simulink model "turtle_waypoint"  (R2017b)
settings: Solver=FixedStepDiscrete  StartTime=0.0  StopTime=inf  FixedStep=0.1  RelTol=1e-3  EnableMultiTasking=on
undefined symbols (not defined in the file): Angular, Linear
libraries: robotlib x3, simulink x1
settings Model: Creator=The MathWorks, Inc.  LastModifiedBy=mraudett
settings DataIOCC: LimitDataPoints=on  SaveFormat=Array
settings OptimizationCC: DefaultUnderspecifiedDataType=single  LifeSpan=1  MaxStackSize=64
settings DebuggingCC: SolverPrmCheckMsg=warning  SFUnexpectedBacktrackingDiag=warning  SFNoUnconditionalDefaultTransitionDiag=warning  SFExecutionAtInitializationDiag=none
settings HardwareCC: ProdBitPerPointer=32  ProdBitPerSizeT=32  ProdBitPerPtrDiffT=32  ProdLargestAtomicFloat=None  ProdIntDivRoundTo=Undefined  ProdEndianess=Unspecified  ProdWordSize=32  ProdHWDeviceType=Generic->Unspecified (assume 32-bit Generic)  TargetHWDeviceType=Generic->Unspecified (assume 32-bit Generic)  UseEmbeddedCoderFeatures=off
settings ModelReferenceCC: PropagateSignalLabelsOutOfModel=off
settings RTWCC: SystemTargetFile=ert.tlc  HardwareBoard=Robot Operating System (ROS)  TLCOptions=-aInlineSetEventsForThisBaseRateFcn=TLC_FALSE -aSuppressMultiTaskScheduler=TLC_FALSE -aRateBasedStepFcn=0  TemplateMakefile=ert_default_tmf  Toolchain=Catkin  TargetLang=C++
settings CodeAppCC: StateflowObjectComments=on
settings ERTTargetCC: MultiwordLength=2048  ERTCustomFileBanners=off  MultiInstanceERTCode=on  CodeInterfacePackaging=C++ class  SupportContinuousTime=on  SupportNonInlinedSFcns=on  RemoveResetFunc=off  SupportVariableSizeSignals=on  ModelStepFunctionPrototypeControlCompliant=off  RootIOFormat=Structure reference  ConvertIfToSwitch=off  SuppressUnreachableDefaultCases=off
settings ConfigComp: CovMetricSettings=dw  CovHtmlReporting=on  CovSaveCumulativeToWorkspaceVar=on  CovSaveSingleToWorkspaceVar=on  CovExternalEMLEnable=off  CovSFcnEnable=off

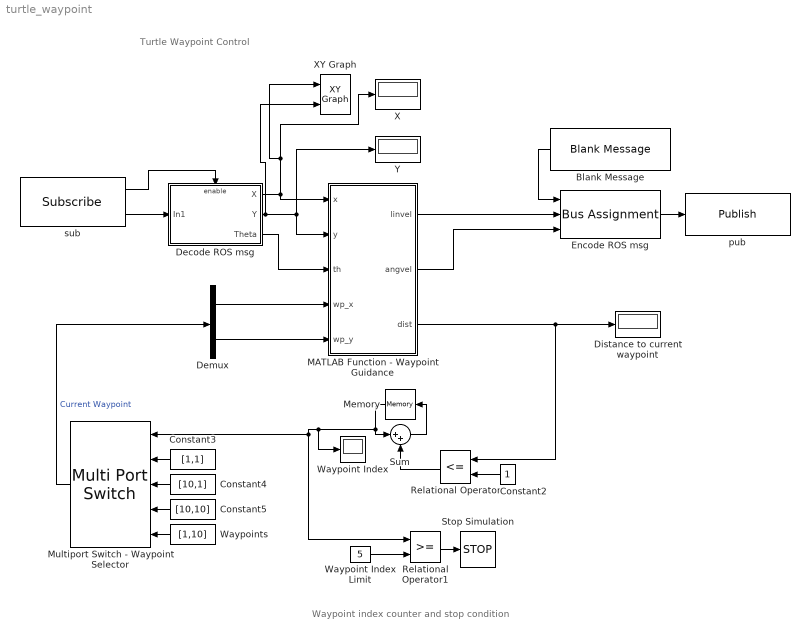
== system turtle_waypoint ==
  note: Waypoint index counter and stop condition
  note: Turtle Waypoint Control
  Blank Message : robotlib/Blank Message  SourceLibraryInfo=This block requires Robotics System Toolbox  messageType=geometry_msgs/Twist  SampleTime=inf
      settings: SourceProductBaseCode=RO
  Constant2 : Constant
  Constant3 : Constant  Value=[1,1]
  Constant4 : Constant  Value=[10,1]
  Constant5 : Constant  Value=[10,10]
  Decode ROS msg : Subsystem
  Demux : Demux  Outputs=2
  Distance to current waypoint : Display
  Encode ROS msg : BusAssignment  AssignedSignals=Linear.X,Angular.Z
  MATLAB Function - Waypoint Guidance : MATLAB Function  TreatAsAtomicUnit=on
  Memory : Memory  InitialCondition=1
  Multiport Switch - Waypoint Selector : MultiPortSwitch  Inputs=4  DiagnosticForDefault=Warning
  Relational Operator : RelationalOperator  Operator=<=  OutDataTypeStr=boolean  RndMeth=Simplest
  Relational Operator1 : RelationalOperator  OutDataTypeStr=boolean  RndMeth=Simplest
  Stop Simulation : Stop
  Sum : Sum  Inputs=|++
  Waypoint Index : Display
  Waypoint Index Limit : Constant  Value=5
  Waypoints : Constant  Value=[1,10]
  X : Display
  XY Graph : simulink/Sinks/XY Graph  xmin=0  xmax=15  ymin=0  ymax=15  st=-1
  Y : Display
  pub : robotlib/Publish  SourceLibraryInfo=This block requires Robotics System Toolbox  topicSource=Specify your own  topic=/turtle1/cmd_vel  messageType=geometry_msgs/Twist  messageQueueLength=105
      settings: SourceProductBaseCode=RO
  "sub " : robotlib/Subscribe  SourceLibraryInfo=This block requires Robotics System Toolbox  topicSource=Specify your own  topic=/turtle1/pose  messageType=turtlesim/Pose  sampleTime=-1  messageQueueLength=51
      settings: SourceProductBaseCode=RO
  wires:
  Encode ROS msg/1 -> pub/1
  "sub "/1 -> Decode ROS msg/Enable
  "sub "/2 -> Decode ROS msg/1(In1)
  Blank Message/1 -> Encode ROS msg/1
  Decode ROS msg/1(X) -> X/1, XY Graph/1, MATLAB Function - Waypoint Guidance/1(x)
  Decode ROS msg/2(Y) -> XY Graph/2, Y/1, MATLAB Function - Waypoint Guidance/2(y)
  Decode ROS msg/3(Theta) -> MATLAB Function - Waypoint Guidance/3(th)
  MATLAB Function - Waypoint Guidance/1(linvel) -> Encode ROS msg/2
  MATLAB Function - Waypoint Guidance/2(angvel) -> Encode ROS msg/3
  MATLAB Function - Waypoint Guidance/3(dist) -> Relational Operator/1, Distance to current waypoint/1
  Constant2/1 -> Relational Operator/2
  Sum/1 -> Memory/1
  Memory/1 -> Waypoint Index/1, Multiport Switch - Waypoint Selector/1, Relational Operator1/1, Sum/1
  Constant3/1 -> Multiport Switch - Waypoint Selector/2
  Demux/1 -> MATLAB Function - Waypoint Guidance/4(wp_x)
  Demux/2 -> MATLAB Function - Waypoint Guidance/5(wp_y)
  Multiport Switch - Waypoint Selector/1 -> Demux/1  "Current Waypoint"
  Constant4/1 -> Multiport Switch - Waypoint Selector/3
  Constant5/1 -> Multiport Switch - Waypoint Selector/4
  Waypoints/1 -> Multiport Switch - Waypoint Selector/5
  Relational Operator/1 -> Sum/2
  Waypoint Index Limit/1 -> Relational Operator1/2
  Relational Operator1/1 -> Stop Simulation/1

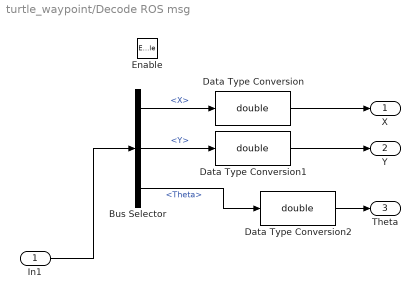
== system turtle_waypoint/Decode ROS msg ==
  In1 : Inport
  Enable : EnablePort
  Bus Selector : BusSelector  DialogController=Simulink.DDGSource_BusSelector  OutputSignals=X,Y,Theta
  Data Type Conversion : DataTypeConversion  OutDataTypeStr=double
  Data Type Conversion1 : DataTypeConversion  OutDataTypeStr=double
  Data Type Conversion2 : DataTypeConversion  OutDataTypeStr=double
  X : Outport
  Y : Outport  Port=2
  Theta : Outport  Port=3
  wires:
  In1/1 -> Bus Selector/1
  Bus Selector/2 -> Data Type Conversion1/1  "<Y>"
  Bus Selector/1 -> Data Type Conversion/1  "<X>"
  Bus Selector/3 -> Data Type Conversion2/1  "<Theta>"
  Data Type Conversion/1 -> X/1
  Data Type Conversion1/1 -> Y/1
  Data Type Conversion2/1 -> Theta/1

== matlab function turtle_waypoint/MATLAB Function - Waypoint Guidance ==
  data: linvel output; angvel output; x input; dist output; y input; th input; wp_x input; wp_y input
function [linvel,angvel,dist] = wpt_fcn(x,y,th,wp_x,wp_y)
% Function to implement waypoint guidance
% Inputs:
%  - x: Current X position
%  - y: Current Y position
%  - th: Current theta position
%  - wp_x: Current waypoint goals, X
%  - wp_y: Current waypoint goals, X
% Outputs:
%  - dist: Distance from current position to current waypoint goal
%  - angvel: Desired angular velocity [rad/s, clockwise]
%  - linvel: Desired linear velocity


% Distance from waypoint to current location
dist = sqrt((x-wp_x)^2+(y-wp_y)^2);

% Angle from current location to waypoint
course = atan2(wp_y-y,wp_x-x);

% Difference (error) between current turtle angle and desired angle
dhdg = course-th;

% Unwrap angle
while dhdg < -pi
    dhdg = dhdg + 2*pi;
end
while dhdg > pi
    dhdg = dhdg - 2*pi;
end

% Proportional Control
% Gains
if dist > 3
    Kpvel = 1.0
else
    Kpvel = 0.5;  % Proportional gain for velocity
end
Kphdg = 10.0;  % Proportional gain for heading

% Specify commands to turtle
angvel=Kphdg*dhdg;
linvel = Kpvel*dist;

end
